simulink model "MVDRBeamformerHDLOptimizedModel"  (R2024b)
settings: Solver=FixedStepDiscrete  StartTime=0.0  StopTime=1.5  RelTol=1e-3
InitFcn:
  | % Initialize signal and noise directions
  | % https://www.mathworks.com/matlabcentral/answers/133622-how-to-change-simulink-constant-block-value-to-a-constant-variable
  | set_param([gcs,'/Noise 1 Direction'],'Value',num2str(30));
  | set_param([gcs,'/Noise 2 Direction'],'Value',num2str(50));
  | set_param([gcs,'/Signal Direction'],'Value',num2str(45));
  | set_param([gcs,'/SteeringAngle'],'Value',num2str(45));
model workspace (MAT data in the model file):
  M = 300
  OutputType : handle (value not decoded)
  T.Input = embedded.fi
  T.Input.DataType = 'Fixed'
  T.Input.Scaling = 'BinaryPoint'
  T.Input.Signed = 1
  T.Input.WordLength = 37
  T.Input.FixedExponent = -24
  T.Input.SlopeAdjustmentFactor = 1
  T.Input.Bias = 0
  T.Input.DataTypeOverride = 'Inherit'
  T.Input.intarray = [0; 0]
  T.Input.noverflows = 0
  T.Input.nunderflows = 0
  T.Input.maxlog = -1.79769313486e+308
  T.Input.minlog = 1.79769313486e+308
  T.Input.RoundingMethod = 'Nearest'
  T.Input.OverflowAction = 'Saturate'
  T.Input.ProductMode = 'FullPrecision'
  T.Input.SumMode = 'FullPrecision'
  T.Input.ProductWordLength = 32
  T.Input.SumWordLength = 32
  T.Input.MaxProductWordLength = 65535
  T.Input.MaxSumWordLength = 65535
  T.Input.ProductFractionLength = 30
  T.Input.ProductFixedExponent = -30
  T.Input.ProductSlope = 9.31322574615e-10
  T.Input.ProductSlopeAdjustmentFactor = 1
  T.Input.ProductBias = 0
  T.Input.SumFractionLength = 30
  T.Input.SumFixedExponent = -30
  T.Input.SumSlope = 9.31322574615e-10
  T.Input.SumSlopeAdjustmentFactor = 1
  T.Input.SumBias = 0
  T.Input.CastBeforeSum = 1
  T.Input.DDGMaxProductWordLength = 65535
  T.Input.DDGMaxSumWordLength = 65535
  T.Input.DDGProductFixedExponent = -30
  T.Input.DDGProductFractionLength = 30
  T.Input.DDGProductWordLength = 32
  T.Input.DDGSumFixedExponent = -30
  T.Input.DDGSumFractionLength = 30
  T.Input.DDGSumWordLength = 32
  T.Input.DDGCastBeforeSum = 1
  T.Input.DDGProductBias = 0
  T.Input.DDGProductSlopeAdjustmentFactor = 1
  T.Input.DDGSumBias = 0
  T.Input.DDGSumSlopeAdjustmentFactor = 1
  T.Input.DDGProductSlope = 9.31322574615e-10
  T.Input.DDGSumSlope = 9.31322574615e-10
  T.Input.Logging = 0
  T.Input.fimathislocal = 0
  T.Output = embedded.fi
  T.Output.DataType = 'Fixed'
  T.Output.Scaling = 'BinaryPoint'
  T.Output.Signed = 1
  T.Output.WordLength = 40
  T.Output.FixedExponent = -24
  T.Output.SlopeAdjustmentFactor = 1
  T.Output.Bias = 0
  T.Output.DataTypeOverride = 'Inherit'
  T.Output.intarray = [0; 0]
  T.Output.noverflows = 0
  T.Output.nunderflows = 0
  T.Output.maxlog = -1.79769313486e+308
  T.Output.minlog = 1.79769313486e+308
  T.Output.RoundingMethod = 'Nearest'
  T.Output.OverflowAction = 'Saturate'
  T.Output.ProductMode = 'FullPrecision'
  T.Output.SumMode = 'FullPrecision'
  T.Output.ProductWordLength = 32
  T.Output.SumWordLength = 32
  T.Output.MaxProductWordLength = 65535
  T.Output.MaxSumWordLength = 65535
  T.Output.ProductFractionLength = 30
  T.Output.ProductFixedExponent = -30
  T.Output.ProductSlope = 9.31322574615e-10
  T.Output.ProductSlopeAdjustmentFactor = 1
  T.Output.ProductBias = 0
  T.Output.SumFractionLength = 30
  T.Output.SumFixedExponent = -30
  T.Output.SumSlope = 9.31322574615e-10
  T.Output.SumSlopeAdjustmentFactor = 1
  T.Output.SumBias = 0
  T.Output.CastBeforeSum = 1
  T.Output.DDGMaxProductWordLength = 65535
  T.Output.DDGMaxSumWordLength = 65535
  T.Output.DDGProductFixedExponent = -30
  T.Output.DDGProductFractionLength = 30
  T.Output.DDGProductWordLength = 32
  T.Output.DDGSumFixedExponent = -30
  T.Output.DDGSumFractionLength = 30
  T.Output.DDGSumWordLength = 32
  T.Output.DDGCastBeforeSum = 1
  T.Output.DDGProductBias = 0
  T.Output.DDGProductSlopeAdjustmentFactor = 1
  T.Output.DDGSumBias = 0
  T.Output.DDGSumSlopeAdjustmentFactor = 1
  T.Output.DDGProductSlope = 9.31322574615e-10
  T.Output.DDGSumSlope = 9.31322574615e-10
  T.Output.Logging = 0
  T.Output.fimathislocal = 0
  T.SteeringVector = embedded.fi
  T.SteeringVector.DataType = 'Fixed'
  T.SteeringVector.Scaling = 'BinaryPoint'
  T.SteeringVector.Signed = 1
  T.SteeringVector.WordLength = 37
  T.SteeringVector.FixedExponent = -35
  T.SteeringVector.SlopeAdjustmentFactor = 1
  T.SteeringVector.Bias = 0
  T.SteeringVector.DataTypeOverride = 'Inherit'
  T.SteeringVector.intarray = [0; 0]
  T.SteeringVector.noverflows = 0
  T.SteeringVector.nunderflows = 0
  T.SteeringVector.maxlog = -1.79769313486e+308
  T.SteeringVector.minlog = 1.79769313486e+308
  T.SteeringVector.RoundingMethod = 'Floor'
  T.SteeringVector.OverflowAction = 'Wrap'
  T.SteeringVector.ProductMode = 'FullPrecision'
  T.SteeringVector.SumMode = 'FullPrecision'
  T.SteeringVector.ProductWordLength = 32
  T.SteeringVector.SumWordLength = 32
  T.SteeringVector.MaxProductWordLength = 65535
  T.SteeringVector.MaxSumWordLength = 65535
  T.SteeringVector.ProductFractionLength = 30
  T.SteeringVector.ProductFixedExponent = -30
  T.SteeringVector.ProductSlope = 9.31322574615e-10
  T.SteeringVector.ProductSlopeAdjustmentFactor = 1
  T.SteeringVector.ProductBias = 0
  T.SteeringVector.SumFractionLength = 30
  T.SteeringVector.SumFixedExponent = -30
  T.SteeringVector.SumSlope = 9.31322574615e-10
  T.SteeringVector.SumSlopeAdjustmentFactor = 1
  T.SteeringVector.SumBias = 0
  T.SteeringVector.CastBeforeSum = 1
  T.SteeringVector.DDGMaxProductWordLength = 65535
  T.SteeringVector.DDGMaxSumWordLength = 65535
  T.SteeringVector.DDGProductFixedExponent = -30
  T.SteeringVector.DDGProductFractionLength = 30
  T.SteeringVector.DDGProductWordLength = 32
  T.SteeringVector.DDGSumFixedExponent = -30
  T.SteeringVector.DDGSumFractionLength = 30
  T.SteeringVector.DDGSumWordLength = 32
  T.SteeringVector.DDGCastBeforeSum = 1
  T.SteeringVector.DDGProductBias = 0
  T.SteeringVector.DDGProductSlopeAdjustmentFactor = 1
  T.SteeringVector.DDGSumBias = 0
  T.SteeringVector.DDGSumSlopeAdjustmentFactor = 1
  T.SteeringVector.DDGProductSlope = 9.31322574615e-10
  T.SteeringVector.DDGSumSlope = 9.31322574615e-10
  T.SteeringVector.Logging = 0
  T.SteeringVector.fimathislocal = 1
  T.ForgettingFactor = embedded.fi
  T.ForgettingFactor.DataType = 'Fixed'
  T.ForgettingFactor.Scaling = 'BinaryPoint'
  T.ForgettingFactor.Signed = 1
  T.ForgettingFactor.WordLength = 37
  T.ForgettingFactor.FixedExponent = -36
  T.ForgettingFactor.SlopeAdjustmentFactor = 1
  T.ForgettingFactor.Bias = 0
  T.ForgettingFactor.DataTypeOverride = 'Inherit'
  T.ForgettingFactor.intarray = [4180530225; 15]
  T.ForgettingFactor.noverflows = 0
  T.ForgettingFactor.nunderflows = 0
  T.ForgettingFactor.maxlog = -1.79769313486e+308
  T.ForgettingFactor.minlog = 1.79769313486e+308
  T.ForgettingFactor.RoundingMethod = 'Nearest'
  T.ForgettingFactor.OverflowAction = 'Saturate'
  T.ForgettingFactor.ProductMode = 'FullPrecision'
  T.ForgettingFactor.SumMode = 'FullPrecision'
  T.ForgettingFactor.ProductWordLength = 32
  T.ForgettingFactor.SumWordLength = 32
  T.ForgettingFactor.MaxProductWordLength = 65535
  T.ForgettingFactor.MaxSumWordLength = 65535
  T.ForgettingFactor.ProductFractionLength = 30
  T.ForgettingFactor.ProductFixedExponent = -30
  T.ForgettingFactor.ProductSlope = 9.31322574615e-10
  T.ForgettingFactor.ProductSlopeAdjustmentFactor = 1
  T.ForgettingFactor.ProductBias = 0
  T.ForgettingFactor.SumFractionLength = 30
  T.ForgettingFactor.SumFixedExponent = -30
  T.ForgettingFactor.SumSlope = 9.31322574615e-10
  T.ForgettingFactor.SumSlopeAdjustmentFactor = 1
  T.ForgettingFactor.SumBias = 0
  T.ForgettingFactor.CastBeforeSum = 1
  T.ForgettingFactor.DDGMaxProductWordLength = 65535
  T.ForgettingFactor.DDGMaxSumWordLength = 65535
  T.ForgettingFactor.DDGProductFixedExponent = -30
  T.ForgettingFactor.DDGProductFractionLength = 30
  T.ForgettingFactor.DDGProductWordLength = 32
  T.ForgettingFactor.DDGSumFixedExponent = -30
  T.ForgettingFactor.DDGSumFractionLength = 30
  T.ForgettingFactor.DDGSumWordLength = 32
  T.ForgettingFactor.DDGCastBeforeSum = 1
  T.ForgettingFactor.DDGProductBias = 0
  T.ForgettingFactor.DDGProductSlopeAdjustmentFactor = 1
  T.ForgettingFactor.DDGSumBias = 0
  T.ForgettingFactor.DDGSumSlopeAdjustmentFactor = 1
  T.ForgettingFactor.DDGProductSlope = 9.31322574615e-10
  T.ForgettingFactor.DDGSumSlope = 9.31322574615e-10
  T.ForgettingFactor.Logging = 0
  T.ForgettingFactor.fimathislocal = 0
  T.M = 300
  forgettingFactor = embedded.fi
  forgettingFactor.DataType = 'Fixed'
  forgettingFactor.Scaling = 'BinaryPoint'
  forgettingFactor.Signed = 1
  forgettingFactor.WordLength = 37
  forgettingFactor.FixedExponent = -36
  forgettingFactor.SlopeAdjustmentFactor = 1
  forgettingFactor.Bias = 0
  forgettingFactor.DataTypeOverride = 'Inherit'
  forgettingFactor.intarray = [4180530225; 15]
  forgettingFactor.noverflows = 0
  forgettingFactor.nunderflows = 0
  forgettingFactor.maxlog = -1.79769313486e+308
  forgettingFactor.minlog = 1.79769313486e+308
  forgettingFactor.RoundingMethod = 'Nearest'
  forgettingFactor.OverflowAction = 'Saturate'
  forgettingFactor.ProductMode = 'FullPrecision'
  forgettingFactor.SumMode = 'FullPrecision'
  forgettingFactor.ProductWordLength = 32
  forgettingFactor.SumWordLength = 32
  forgettingFactor.MaxProductWordLength = 65535
  forgettingFactor.MaxSumWordLength = 65535
  forgettingFactor.ProductFractionLength = 30
  forgettingFactor.ProductFixedExponent = -30
  forgettingFactor.ProductSlope = 9.31322574615e-10
  forgettingFactor.ProductSlopeAdjustmentFactor = 1
  forgettingFactor.ProductBias = 0
  forgettingFactor.SumFractionLength = 30
  forgettingFactor.SumFixedExponent = -30
  forgettingFactor.SumSlope = 9.31322574615e-10
  forgettingFactor.SumSlopeAdjustmentFactor = 1
  forgettingFactor.SumBias = 0
  forgettingFactor.CastBeforeSum = 1
  forgettingFactor.DDGMaxProductWordLength = 65535
  forgettingFactor.DDGMaxSumWordLength = 65535
  forgettingFactor.DDGProductFixedExponent = -30
  forgettingFactor.DDGProductFractionLength = 30
  forgettingFactor.DDGProductWordLength = 32
  forgettingFactor.DDGSumFixedExponent = -30
  forgettingFactor.DDGSumFractionLength = 30
  forgettingFactor.DDGSumWordLength = 32
  forgettingFactor.DDGCastBeforeSum = 1
  forgettingFactor.DDGProductBias = 0
  forgettingFactor.DDGProductSlopeAdjustmentFactor = 1
  forgettingFactor.DDGSumBias = 0
  forgettingFactor.DDGSumSlopeAdjustmentFactor = 1
  forgettingFactor.DDGProductSlope = 9.31322574615e-10
  forgettingFactor.DDGSumSlope = 9.31322574615e-10
  forgettingFactor.Logging = 0
  forgettingFactor.fimathislocal = 0
  nArrayElements = 10
  noise1Variance = 100
  noise2Variance = 100
  paramBeamformerI.propSpeed = 299792458
  paramBeamformerI.fc = 100000000
  paramBeamformerI.Antenna = phased.ULA
  paramBeamformerI.Antenna.any.ClassNameForLoadTimeEval = 'phased.ULA'
  paramBeamformerI.Antenna.any.MajorVersionNumber = 24
  paramBeamformerI.Antenna.any.MinorVersionNumber = 512
  paramBeamformerI.Antenna.any.ChildClassData.NumElements = 10
  paramBeamformerI.Antenna.any.ChildClassData.ElementSpacing = 1.49896229
  paramBeamformerI.Antenna.any.ChildClassData.ArrayAxis = 'y'
  paramBeamformerI.Antenna.any.ChildClassData.Taper = 1
  paramBeamformerI.Antenna.any.ChildClassData.Element.ClassNameForLoadTimeEval = 'phased.IsotropicAntennaElement'
  paramBeamformerI.Antenna.any.ChildClassData.Element.MajorVersionNumber = 24
  paramBeamformerI.Antenna.any.ChildClassData.Element.MinorVersionNumber = 512
  paramBeamformerI.Antenna.any.ChildClassData.Element.ChildClassData.FrequencyRange = [0 1e+20]
  paramBeamformerI.Antenna.any.ChildClassData.Element.ChildClassData.BackBaffled = 0
  paramBeamformerI.Antenna.any.ChildClassData.Element.ChildClassData.pOutputCombinedPattern = 0
  paramBeamformerI.Antenna.any.ChildClassData.Element.ChildClassData.pIsOutputComplex = 1
  paramBeamformerI.Antenna.any.ChildClassData.Element.SuperClassData = []
  paramBeamformerI.Antenna.any.ChildClassData.isLocked = 0
  paramBeamformerI.Antenna.any.SuperClassData = []
  paramBeamformerI.fs = 1000
  paramBeamformerI.prf = 3.33333333333
  paramBeamformerI.samplesPerFrame = 1
  paramBeamformerI.cMatrix = [-0.976602248144+0.21505359546i  -0.840977704306+0.541069774485i  -0.61019358433+0.792252352248i; 0.347607244607-0.937640231377i  0.0788545425829-0.996886132472i  -0.186572596413-0.982441177001i; 0.600409925306+0.799692391857i  0.745453332383+0.666557821377i  0.858147047038+0.513403979006i; -0.997391183118+0.0721860640226i  -0.981896511259+0.189418164855i  -0.953897847357+0.300131465873i; 0.479000563904-0.877814593055i  0.444015840326-0.896018935927i  0.409575431342-0.912276255331i; 0.479000563904+0.877814593055i  0.444015840326+0.896018935927i  0.409575431342+0.912276255331i; -0.997391183118-0.0721860640226i  -0.981896511259-0.189418164855i  -0.953897847357-0.300131465873i; 0.600409925306-0.799692391857i  0.745453332383-0.666557821377i  0.858147047038-0.513403979006i; 0.347607244607+0.937640231377i  0.0788545425829+0.996886132472i  -0.186572596413+0.982441177001i; -0.976602248144-0.21505359546i  -0.840977704306-0.541069774485i  -0.61019358433-0.792252352248i]
  pulseMagnitude = 1
  qlessQRCyclesToReady = 46
  samplesPerFrame = 300
  thermalNoisePower = 1e-05
values from neighbouring files (symbols this model uses):
  paramBeamformerI = beamformerParameters(nArrayElements)    [setMVDRExampleModelWorkspace.m]
  T = mvdr_types('Fixed',m,nArrayElements,pulseMagnitude,thermalNoisePower,noise1Variance,noise2Variance)    [setMVDRExampleModelWorkspace.m]
undefined symbols (not defined in the file or in its folder): physconst
libraries: dspsigops x5, phasedtxrxlib x3, dspobslib x2, embsystolicmatrixops x1, embreciprocals x1, phasedwavlib x1
settings Model: DataTypeOverride=Off  SimulationMode=accelerator  Creator=The MathWorks, Inc.  LastModifiedBy=The MathWorks, Inc.
settings SolverCC: AlgebraicLoopSolver=TrustRegion  MaxZcPerStep=1
settings DataIOCC: SaveOutput=off  SignalLogging=off  SaveTime=off
settings OptimizationCC: BlockReduction=off  ConditionallyExecuteInputs=off  DefaultParameterBehavior=Inlined  ReuseModelBlockBuffer=off
settings DebuggingCC: AlgebraicLoopMsg=error  SingleTaskRateTransMsg=error  ParameterDowncastMsg=none  ParameterOverflowMsg=none  ParameterPrecisionLossMsg=none  ParameterTunabilityLossMsg=none  FixptConstOverflowMsg=warning  UnconnectedInputMsg=warning  UnconnectedOutputMsg=warning  UnconnectedLineMsg=warning
settings HardwareCC: ProdBitPerPointer=32  ProdBitPerSizeT=32  ProdBitPerPtrDiffT=32  ProdLargestAtomicFloat=None  ProdIntDivRoundTo=Undefined  ProdEndianess=Unspecified  ProdWordSize=32  ProdHWDeviceType=ASIC/FPGA->ASIC/FPGA  TargetBitPerLong=64  TargetBitPerPointer=64  TargetBitPerSizeT=64  TargetBitPerPtrDiffT=64  TargetLongLongMode=on  TargetIntDivRoundTo=Zero  TargetEndianess=LittleEndian  TargetWordSize=64  TargetHWDeviceType=Custom Processor->MATLAB Host Computer  ProdEqTarget=off
settings ModelReferenceCC: EnableRefExpFcnMdlSchedulingChecks=on
settings RTWCC: GPUComputeCapability=3.5  DLArmComputeVersion=19.05

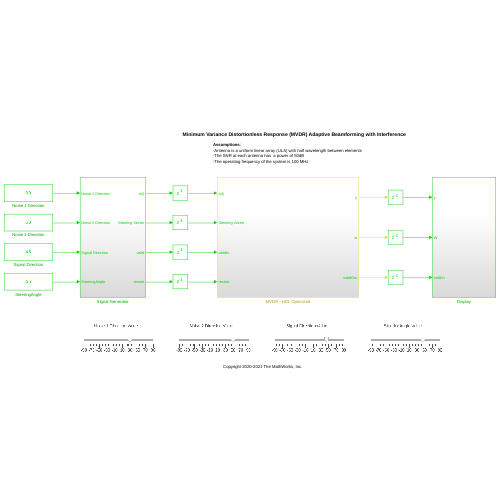
[thumbnail: Simulink's stored preview of the top-level diagram]
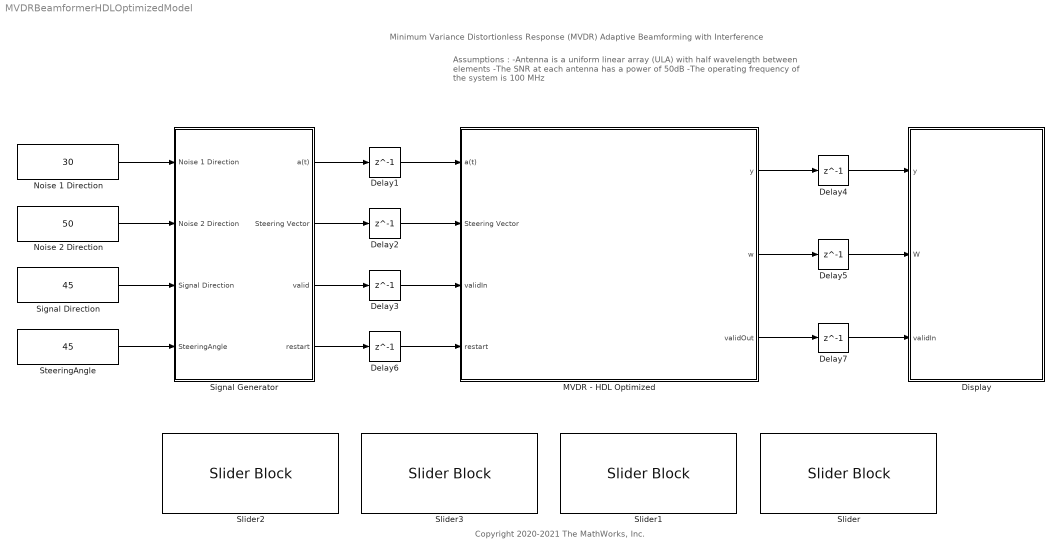
== system MVDRBeamformerHDLOptimizedModel ==
  note: Copyright 2020-2021 The MathWorks, Inc.
  note: Minimum Variance Distortionless Response (MVDR) Adaptive Beamforming with Interference
  note: Assumptions :
      | -Antenna is a uniform linear array (ULA) with half wavelength between elements
      | -The SNR at each antenna has a power of 50dB
      | -The operating frequency of the system is 100 MHz
  Delay{1..7} (7 alike) : Delay  DelayLength=1
  Display : Subsystem
  MVDR - HDL Optimized : Subsystem
  Noise 1 Direction : Constant  Value=30  VectorParams1D=off  SampleTime=-1
  Noise 2 Direction : Constant  Value=50  VectorParams1D=off  SampleTime=-1
  Signal Direction : Constant  Value=45  VectorParams1D=off  SampleTime=-1
  Signal Generator : Subsystem
  Slider{,1..3} (4 alike) : SliderBlock  ScaleMin=-90  ScaleMax=90
  SteeringAngle : Constant  Value=45  VectorParams1D=off  SampleTime=-1
  wires:
  MVDR - HDL Optimized/3(validOut) -> Delay7/1
  Delay3/1 -> MVDR - HDL Optimized/3(validIn)
  Delay4/1 -> Display/1(y)
  Signal Generator/3(valid) -> Delay3/1
  Noise 1 Direction/1 -> Signal Generator/1(Noise 1 Direction)
  Noise 2 Direction/1 -> Signal Generator/2(Noise 2 Direction)
  Signal Generator/2(Steering Vector) -> Delay2/1
  Signal Generator/4(restart) -> Delay6/1
  MVDR - HDL Optimized/1(y) -> Delay4/1
  SteeringAngle/1 -> Signal Generator/4(SteeringAngle)
  Delay5/1 -> Display/2(W)
  Signal Direction/1 -> Signal Generator/3(Signal Direction)
  MVDR - HDL Optimized/2(w) -> Delay5/1
  Delay1/1 -> MVDR - HDL Optimized/1(a(t))
  Signal Generator/1(a(t)) -> Delay1/1
  Delay2/1 -> MVDR - HDL Optimized/2(Steering Vector)
  Delay7/1 -> Display/3(validIn)
  Delay6/1 -> MVDR - HDL Optimized/4(restart)

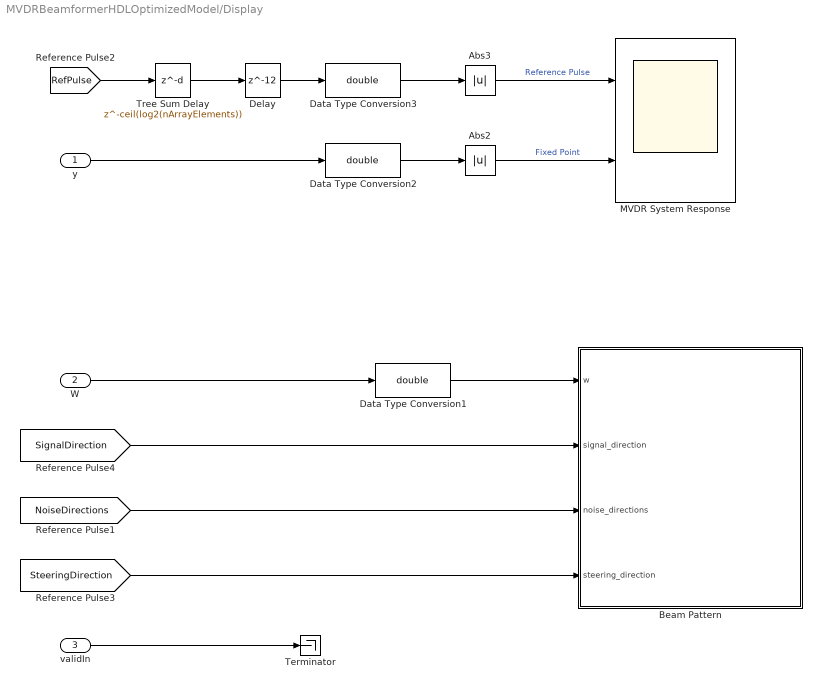
== system MVDRBeamformerHDLOptimizedModel/Display ==
  y : Inport
  W : Inport  Port=2
  validIn : Inport  Port=3
  Abs2 : Abs  SaturateOnIntegerOverflow=off
  Abs3 : Abs  SaturateOnIntegerOverflow=off
  Beam Pattern : MATLAB Function  TreatAsAtomicUnit=on  mask{M=M, nArrayElements=nArrayElements}
      mask prompts: nArrayElements "Number of array elements"
  Data Type Conversion1 : DataTypeConversion  OutDataTypeStr=double  SaturateOnIntegerOverflow=off  RndMeth=Floor
  Data Type Conversion2 : DataTypeConversion  OutDataTypeStr=double  SaturateOnIntegerOverflow=off  RndMeth=Floor
  Data Type Conversion3 : DataTypeConversion  OutDataTypeStr=double  SaturateOnIntegerOverflow=off  RndMeth=Floor
  Delay : Delay  DelayLength=12
  MVDR System Response : Scope  NumInputPorts=2
  Terminator : Terminator
  Tree Sum Delay : Delay  DelayLength=ceil(log2(nArrayElements))
  wires:
  Abs3/1 -> MVDR System Response/1  "Reference Pulse"
  Abs2/1 -> MVDR System Response/2  "Fixed Point"
  y/1 -> Data Type Conversion2/1
  Data Type Conversion2/1 -> Abs2/1
  Data Type Conversion3/1 -> Abs3/1
  [SteeringDirection] -> Beam Pattern/4(steering_direction)
  [NoiseDirections] -> Beam Pattern/3(noise_directions)
  [SignalDirection] -> Beam Pattern/2(signal_direction)
  Data Type Conversion1/1 -> Beam Pattern/1(w)
  W/1 -> Data Type Conversion1/1
  [RefPulse] -> Tree Sum Delay/1
  Delay/1 -> Data Type Conversion3/1
  validIn/1 -> Terminator/1
  Tree Sum Delay/1 -> Delay/1

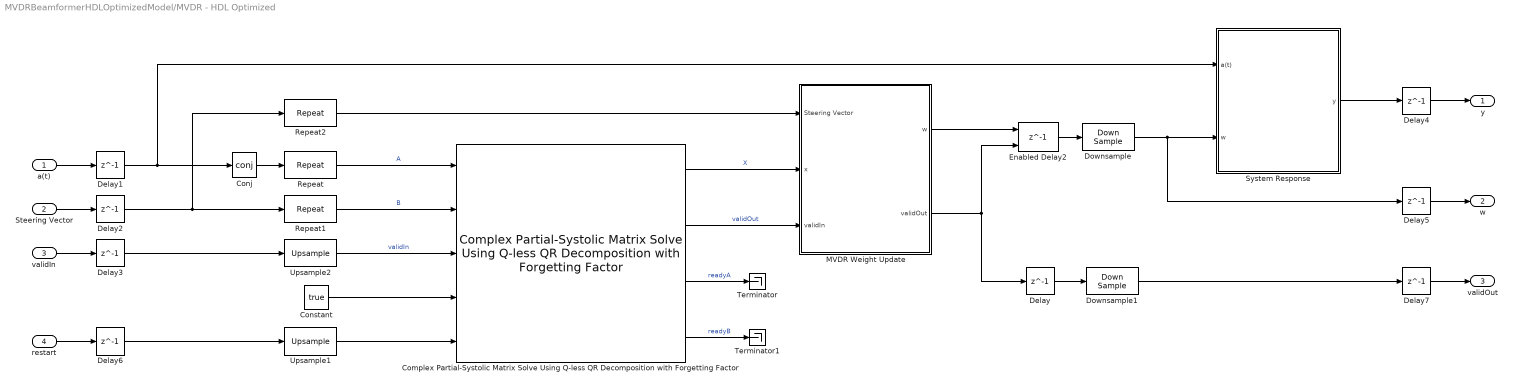
== system MVDRBeamformerHDLOptimizedModel/MVDR - HDL Optimized ==
  a(t) : Inport
  Steering Vector : Inport  Port=2
  validIn : Inport  Port=3
  restart : Inport  Port=4
  Complex Partial-Systolic Matrix Solve Using Q-less QR Decomposition with Forgetting Factor : embsystolicmatrixops/Complex Partial-Systolic Matrix Solve Using Q-less QR Decomposition with Forgetting Factor  n=nArrayElements  p=1  forgettingFactor=forgettingFactor  regularizationParameter=0  OutputType=OutputType
  Conj : Math  Operator=conj
  Constant : Constant  Value=true  OutDataTypeStr=boolean  SampleTime=-1
  Delay{,1..7} (8 alike) : Delay  DelayLength=1
  Downsample : DownSample  N=qlessQRCyclesToReady  RateOptions=Allow multirate processing
  Downsample1 : DownSample  N=qlessQRCyclesToReady  RateOptions=Allow multirate processing
  Enabled Delay2 : Delay  DelayLength=1  ShowEnablePort=on
      settings: InputPortMap=u0,e6
  MVDR Weight Update : Subsystem
  Repeat : dspsigops/Repeat  FactorSource=Dialog parameter  N=qlessQRCyclesToReady  Nmax=16  RateOptions=Allow multirate processing  ic=0  mode=Unused parameter value
  Repeat1 : dspsigops/Repeat  FactorSource=Dialog parameter  N=qlessQRCyclesToReady  Nmax=16  RateOptions=Allow multirate processing  ic=0  mode=Unused parameter value
  Repeat2 : dspsigops/Repeat  FactorSource=Dialog parameter  N=qlessQRCyclesToReady  Nmax=16  RateOptions=Allow multirate processing  ic=0  mode=Unused parameter value
  System Response : Subsystem
  Terminator : Terminator
  Terminator1 : Terminator
  Upsample1 : dspsigops/Upsample  FactorSource=Dialog parameter  N=qlessQRCyclesToReady  Nmax=16  phase=0  RateOptions=Allow multirate processing  ic=0  mode=Unused parameter value
  Upsample2 : dspsigops/Upsample  FactorSource=Dialog parameter  N=qlessQRCyclesToReady  Nmax=16  phase=0  RateOptions=Allow multirate processing  ic=0  mode=Unused parameter value
  y : Outport
  w : Outport  Port=2
  validOut : Outport  Port=3
  wires:
  System Response/1(y) -> Delay4/1
  Steering Vector/1 -> Delay2/1
  MVDR Weight Update/2(validOut) -> Delay/1, Enabled Delay2/2
  Complex Partial-Systolic Matrix Solve Using Q-less QR Decomposition with Forgetting Factor/4 -> Terminator1/1  "readyB"
  Complex Partial-Systolic Matrix Solve Using Q-less QR Decomposition with Forgetting Factor/1 -> MVDR Weight Update/2(x)  "X"
  Conj/1 -> Repeat/1
  Delay3/1 -> Upsample2/1
  MVDR Weight Update/1(w) -> Enabled Delay2/1
  Repeat1/1 -> Complex Partial-Systolic Matrix Solve Using Q-less QR Decomposition with Forgetting Factor/2  "B"
  Repeat/1 -> Complex Partial-Systolic Matrix Solve Using Q-less QR Decomposition with Forgetting Factor/1  "A"
  a(t)/1 -> Delay1/1
  validIn/1 -> Delay3/1
  Complex Partial-Systolic Matrix Solve Using Q-less QR Decomposition with Forgetting Factor/3 -> Terminator/1  "readyA"
  Upsample2/1 -> Complex Partial-Systolic Matrix Solve Using Q-less QR Decomposition with Forgetting Factor/3  "validIn"
  Delay2/1 -> Repeat2/1, Repeat1/1
  Delay4/1 -> y/1
  Delay5/1 -> w/1
  Repeat2/1 -> MVDR Weight Update/1(Steering Vector)
  Delay1/1 -> System Response/1(a(t)), Conj/1
  Enabled Delay2/1 -> Downsample/1
  Downsample/1 -> System Response/2(w), Delay5/1
  restart/1 -> Delay6/1
  Delay6/1 -> Upsample1/1
  Upsample1/1 -> Complex Partial-Systolic Matrix Solve Using Q-less QR Decomposition with Forgetting Factor/5
  Downsample1/1 -> Delay7/1
  Complex Partial-Systolic Matrix Solve Using Q-less QR Decomposition with Forgetting Factor/2 -> MVDR Weight Update/3(validIn)  "validOut"
  Delay/1 -> Downsample1/1
  Delay7/1 -> validOut/1
  Constant/1 -> Complex Partial-Systolic Matrix Solve Using Q-less QR Decomposition with Forgetting Factor/4

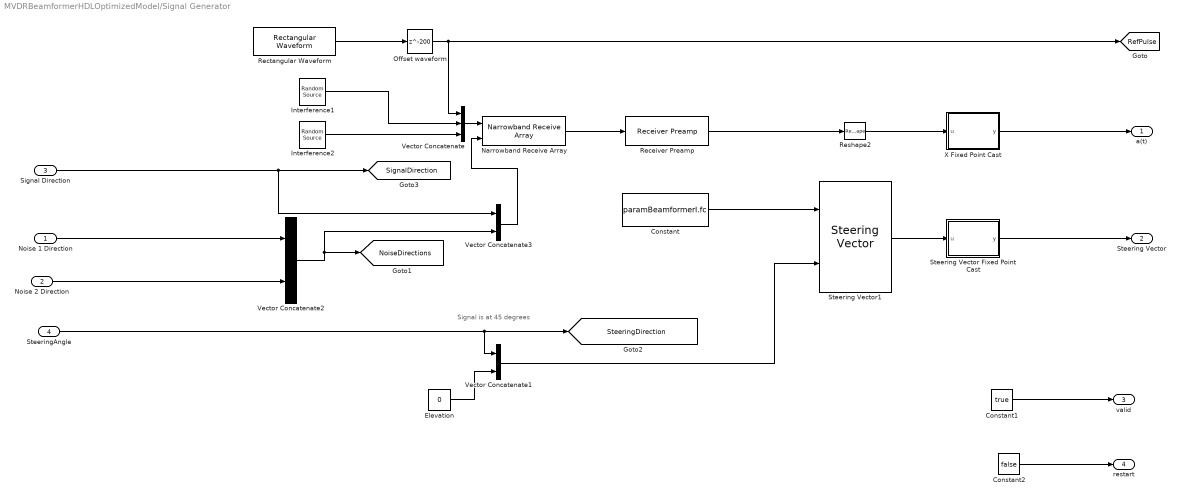
== system MVDRBeamformerHDLOptimizedModel/Signal Generator ==
  note: Signal is at 45 degrees
  Noise 1 Direction : Inport
  Noise 2 Direction : Inport  Port=2
  Signal Direction : Inport  Port=3
  SteeringAngle : Inport  Port=4
  Constant : Constant  Value=paramBeamformerI.fc
  Constant1 : Constant  Value=true  SampleTime=-1
  Constant2 : Constant  Value=false  SampleTime=-1
  Elevation : Constant  Value=0
  Interference1 : dspobslib/Random Source  SrcType=Gaussian  NormMethod=Ziggurat  CltLength=12  MinVal=0  MaxVal=1  MeanVal=0  VarVal=noise1Variance  RepMode=Repeatable  rawSeed=1  IsInherit=off  SampMode=Discrete  SampTime=1/paramBeamformerI.fs  SampFrame=paramBeamformerI.samplesPerFrame  DataType=Double  OutComplex=Real  OutputFrames=on
  Interference2 : dspobslib/Random Source  SrcType=Gaussian  NormMethod=Ziggurat  CltLength=12  MinVal=0  MaxVal=1  MeanVal=0  VarVal=noise2Variance  RepMode=Repeatable  rawSeed=1  IsInherit=off  SampMode=Discrete  SampTime=1/paramBeamformerI.fs  SampFrame=paramBeamformerI.samplesPerFrame  DataType=Double  OutComplex=Real  OutputFrames=on
  Narrowband Receive Array : phasedtxrxlib/Narrowband Receive Array  PropagationSpeed=paramBeamformerI.propSpeed  OperatingFrequency=paramBeamformerI.fc  Wavefront=Plane  SensorGainMeasure=dB  Polarization=None  WeightsInputPort=off  SimulateUsing=Interpreted execution  Sensor=paramBeamformerI.Antenna
  Offset waveform : Delay  DelayLength=200  InputProcessing=Columns as channels (frame based)
  Receiver Preamp : phasedtxrxlib/Receiver Preamp  Gain=0  LossFactor=0  NoiseMethod=Noise power  NoiseFigure=0  ReferenceTemperature=290  SampleRateFromInputCheckbox=on  SampleRate=1e6  NoisePower=thermalNoisePower  EnableInputPort=off  PhaseNoiseInputPort=off  SeedSource=Auto  Seed=0  SimulateUsing=Code generation
  Rectangular Waveform : phasedwavlib/Rectangular Waveform  SampleRate=paramBeamformerI.fs  DurationSpecification=Pulse width  PulseWidth=5/paramBeamformerI.fs  DutyCycle=0.5  PRF=paramBeamformerI.prf  PRFSelectionInputPort=off  SimulationTimeSource=Derive from waveform parameters  FrequencyOffsetSource=Property  FrequencyOffset=0  OutputFormat=Samples  NumSamples=1  NumPulses=1  PRFOutputPort=off  CoefficientsOutputPort=off  SimulateUsing=Interpreted execution
  Reshape2 : Reshape  OutputDimensionality=Column vector (2-D)
  Steering Vector Fixed Point Cast : MATLAB Function  TreatAsAtomicUnit=on  mask{T=T.SteeringVector}
      mask prompts: T "Like parameter"
  Steering Vector1 : phasedtxrxlib/Steering Vector  PropagationSpeed=physconst( 'LightSpeed' )  FrequencySource=Input port  OperatingFrequency=3e8  OutputConjugate=off  NumPhaseShifterBits=0  IncludeElementResponse=off  EnablePolarization=off  SimulateUsing=Code generation  SensorArray=paramBeamformerI.Antenna
  Vector Concatenate : Concatenate  NumInputs=3  Mode=Multidimensional array  ConcatenateDimension=2
  Vector Concatenate1 : Concatenate  Mode=Multidimensional array
  Vector Concatenate2 : Concatenate  Mode=Multidimensional array  ConcatenateDimension=2
  Vector Concatenate3 : Concatenate  Mode=Multidimensional array  ConcatenateDimension=2
  X Fixed Point Cast : MATLAB Function  TreatAsAtomicUnit=on  mask{T=T.Input}
      mask prompts: T "Like parameter"
  a(t) : Outport  VectorParamsAs1DForOutWhenUnconnected=off
  Steering Vector : Outport  Port=2  VectorParamsAs1DForOutWhenUnconnected=off
  valid : Outport  Port=3  PortDimensions=1  VectorParamsAs1DForOutWhenUnconnected=off  LockScale=on
  restart : Outport  Port=4  PortDimensions=1  VectorParamsAs1DForOutWhenUnconnected=off  LockScale=on
  tag scope: NoiseDirections=global, RefPulse=global, SignalDirection=global, SteeringDirection=global
  wires:
  Vector Concatenate3/1 -> Narrowband Receive Array/2
  Interference1/1 -> Vector Concatenate/2
  Interference2/1 -> Vector Concatenate/3
  Elevation/1 -> Vector Concatenate1/2
  Vector Concatenate2/1 -> Vector Concatenate3/2, [NoiseDirections]
  Rectangular Waveform/1 -> Offset waveform/1
  Vector Concatenate/1 -> Narrowband Receive Array/1
  Offset waveform/1 -> [RefPulse], Vector Concatenate/1
  Narrowband Receive Array/1 -> Receiver Preamp/1
  Constant/1 -> Steering Vector1/1
  Vector Concatenate1/1 -> Steering Vector1/2
  Steering Vector1/1 -> Steering Vector Fixed Point Cast/1(u)
  Steering Vector Fixed Point Cast/1(y) -> Steering Vector/1
  Reshape2/1 -> X Fixed Point Cast/1(u)
  X Fixed Point Cast/1(y) -> a(t)/1
  Receiver Preamp/1 -> Reshape2/1
  Signal Direction/1 -> Vector Concatenate3/1, [SignalDirection]
  Noise 1 Direction/1 -> Vector Concatenate2/1
  Noise 2 Direction/1 -> Vector Concatenate2/2
  SteeringAngle/1 -> Vector Concatenate1/1, [SteeringDirection]
  Constant1/1 -> valid/1
  Constant2/1 -> restart/1

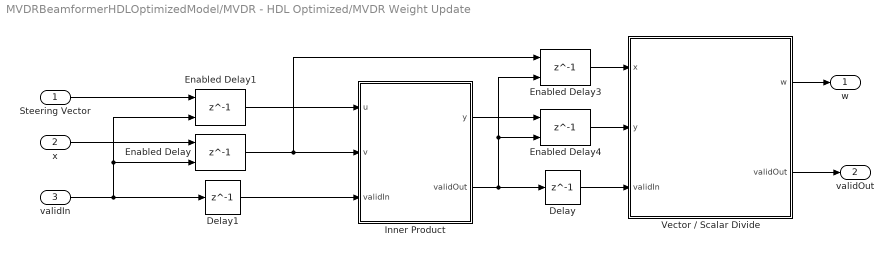
== system MVDRBeamformerHDLOptimizedModel/MVDR - HDL Optimized/MVDR Weight Update ==
  Steering Vector : Inport
  x : Inport  Port=2
  validIn : Inport  Port=3
  Delay : Delay  DelayLength=1
  Delay1 : Delay  DelayLength=1
  Enabled Delay{,1,3..4} (4 alike) : Delay  DelayLength=1  ShowEnablePort=on
      settings: InputPortMap=u0,e6
  Inner Product : Subsystem  mask{n=nArrayElements}
      mask prompts: n "Vector length"
  Vector / Scalar Divide : Subsystem
  w : Outport
  validOut : Outport  Port=2
  wires:
  x/1 -> Enabled Delay/1
  Vector / Scalar Divide/1(w) -> w/1
  Enabled Delay1/1 -> Inner Product/1(u)
  Inner Product/1(y) -> Enabled Delay4/1
  Enabled Delay3/1 -> Vector / Scalar Divide/1(x)
  Delay/1 -> Vector / Scalar Divide/3(validIn)
  Steering Vector/1 -> Enabled Delay1/1
  Enabled Delay/1 -> Enabled Delay3/1, Inner Product/2(v)
  Enabled Delay4/1 -> Vector / Scalar Divide/2(y)
  Inner Product/2(validOut) -> Enabled Delay4/2, Enabled Delay3/2, Delay/1
  validIn/1 -> Enabled Delay1/2, Enabled Delay/2, Delay1/1
  Vector / Scalar Divide/2(validOut) -> validOut/1
  Delay1/1 -> Inner Product/3(validIn)

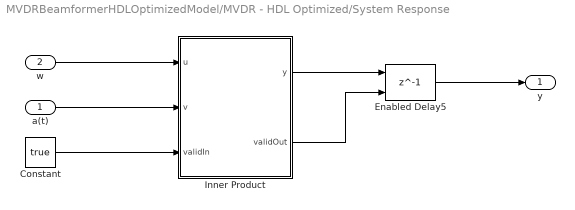
== system MVDRBeamformerHDLOptimizedModel/MVDR - HDL Optimized/System Response ==
  a(t) : Inport
  w : Inport  Port=2
  Constant : Constant  Value=true  SampleTime=-1
  Enabled Delay5 : Delay  DelayLength=1  ShowEnablePort=on
      settings: InputPortMap=u0,e6
  Inner Product : Subsystem  mask{n=nArrayElements}
      mask prompts: n "Vector length"
  y : Outport
  wires:
  Enabled Delay5/1 -> y/1
  a(t)/1 -> Inner Product/2(v)
  Inner Product/2(validOut) -> Enabled Delay5/2
  Constant/1 -> Inner Product/3(validIn)
  Inner Product/1(y) -> Enabled Delay5/1
  w/1 -> Inner Product/1(u)

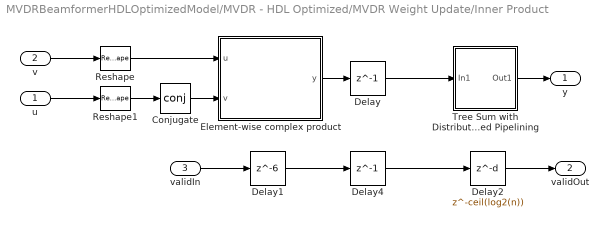
== system MVDRBeamformerHDLOptimizedModel/MVDR - HDL Optimized/MVDR Weight Update/Inner Product ==
  u : Inport
  v : Inport  Port=2
  validIn : Inport  Port=3
  Conjugate : Math  Operator=conj  SignedPower=on  RndMeth=Zero
  Delay : Delay  DelayLength=1
  Delay1 : Delay  DelayLength=6
  Delay2 : Delay  DelayLength=ceil(log2(n))
  Delay4 : Delay  DelayLength=1
  Element-wise complex product : Subsystem  TreatAsAtomicUnit=on
  Reshape : Reshape  OutputDimensionality=Column vector (2-D)
  Reshape1 : Reshape  OutputDimensionality=Column vector (2-D)
  Tree Sum with Distributed Pipelining : Subsystem
  y : Outport
  validOut : Outport  Port=2
  wires:
  v/1 -> Reshape/1
  u/1 -> Reshape1/1
  validIn/1 -> Delay1/1
  Element-wise complex product/1(y) -> Delay/1
  Delay2/1 -> validOut/1
  Delay1/1 -> Delay4/1
  Delay4/1 -> Delay2/1
  Reshape/1 -> Element-wise complex product/1(u)
  Delay/1 -> Tree Sum with Distributed Pipelining/1(In1)
  Tree Sum with Distributed Pipelining/1(Out1) -> y/1
  Reshape1/1 -> Conjugate/1
  Conjugate/1 -> Element-wise complex product/2(v)

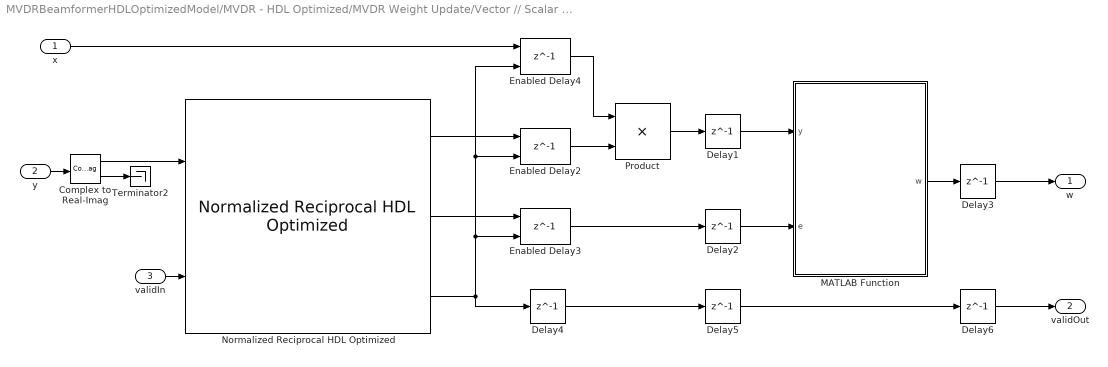
== system MVDRBeamformerHDLOptimizedModel/MVDR - HDL Optimized/MVDR Weight Update/Vector // Scalar Divide ==
  x : Inport
  y : Inport  Port=2
  validIn : Inport  Port=3
  Complex to Real-Imag : ComplexToRealImag
  Delay{1..6} (6 alike) : Delay  DelayLength=1
  Enabled Delay2 : Delay  DelayLength=1  ShowEnablePort=on
      settings: InputPortMap=u0,e6
  Enabled Delay3 : Delay  DelayLength=1  ShowEnablePort=on
      settings: InputPortMap=u0,e6
  Enabled Delay4 : Delay  DelayLength=1  ShowEnablePort=on
      settings: InputPortMap=u0,e6
  MATLAB Function : MATLAB Function  TreatAsAtomicUnit=on
  Normalized Reciprocal HDL Optimized : embreciprocals/Normalized Reciprocal HDL Optimized  dbzPort=off  autoMaximumShiftVal=on  maximumShiftValue=10  nIterPerReg=1
  Product : Product  OutDataTypeStr=Inherit: Same as first input
  Terminator2 : Terminator
  w : Outport
  validOut : Outport  Port=2
  wires:
  Delay2/1 -> MATLAB Function/2(e)
  y/1 -> Complex to Real-Imag/1
  Enabled Delay2/1 -> Product/2
  Complex to Real-Imag/1 -> Normalized Reciprocal HDL Optimized/1
  Enabled Delay4/1 -> Product/1
  Normalized Reciprocal HDL Optimized/2 -> Enabled Delay3/1
  Normalized Reciprocal HDL Optimized/1 -> Enabled Delay2/1
  Delay1/1 -> MATLAB Function/1(y)
  validIn/1 -> Normalized Reciprocal HDL Optimized/2
  Product/1 -> Delay1/1
  Enabled Delay3/1 -> Delay2/1
  MATLAB Function/1(w) -> Delay3/1
  Complex to Real-Imag/2 -> Terminator2/1
  x/1 -> Enabled Delay4/1
  Normalized Reciprocal HDL Optimized/3 -> Delay4/1, Enabled Delay3/2, Enabled Delay4/2, Enabled Delay2/2
  Delay3/1 -> w/1
  Delay4/1 -> Delay5/1
  Delay5/1 -> Delay6/1
  Delay6/1 -> validOut/1

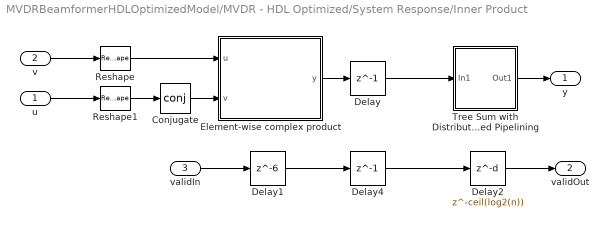
== system MVDRBeamformerHDLOptimizedModel/MVDR - HDL Optimized/System Response/Inner Product ==
  u : Inport
  v : Inport  Port=2
  validIn : Inport  Port=3
  Conjugate : Math  Operator=conj  SignedPower=on  RndMeth=Zero
  Delay : Delay  DelayLength=1
  Delay1 : Delay  DelayLength=6
  Delay2 : Delay  DelayLength=ceil(log2(n))
  Delay4 : Delay  DelayLength=1
  Element-wise complex product : Subsystem  TreatAsAtomicUnit=on
  Reshape : Reshape  OutputDimensionality=Column vector (2-D)
  Reshape1 : Reshape  OutputDimensionality=Column vector (2-D)
  Tree Sum with Distributed Pipelining : Subsystem
  y : Outport
  validOut : Outport  Port=2
  wires:
  v/1 -> Reshape/1
  u/1 -> Reshape1/1
  validIn/1 -> Delay1/1
  Element-wise complex product/1(y) -> Delay/1
  Delay2/1 -> validOut/1
  Delay1/1 -> Delay4/1
  Delay4/1 -> Delay2/1
  Reshape/1 -> Element-wise complex product/1(u)
  Delay/1 -> Tree Sum with Distributed Pipelining/1(In1)
  Tree Sum with Distributed Pipelining/1(Out1) -> y/1
  Reshape1/1 -> Conjugate/1
  Conjugate/1 -> Element-wise complex product/2(v)

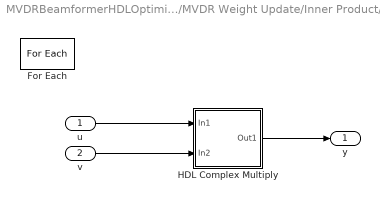
== system MVDRBeamformerHDLOptimizedModel/MVDR - HDL Optimized/MVDR Weight Update/Inner Product/Element-wise complex product ==
  u : Inport  Partition=on  PartitionDimension=1  PartitionWidth=1  PartitionOffset=0
  v : Inport  Port=2  Partition=on  PartitionDimension=1  PartitionWidth=1  PartitionOffset=0
  For Each : ForEach  DisableCoverage=on
  HDL Complex Multiply : Subsystem  mask(HDL Complex Multiplier (3 Multiply, 5 Add)){D1=2, D2=1, D3=1, D4=1, D5=1}
      mask help:
      | Xilinx devices:
      | - Set D1 = 1 or 2 to trade off speed & FF resources
      | - Set D2-D5 = 1 to fully leverage DSP48 pipelines
      | - Use sync reset
      |
      | Intel FPGAs:
      | - Set D1 = 1 or 2 depending on device family
      | - Set D5 = 1; D2, D3, D4 = 0
      | - Use async reset
      mask init:
      | delay = D1+D2+D3+D4+D5;
      mask Display:
      | fprintf('Delay=%d',delay);
      | port_label('input',1,'z1');
      | port_label('input',2,'z2');
  y : Outport  ConcatenationDimension=1
  wires:
  v/1 -> HDL Complex Multiply/2(In2)
  HDL Complex Multiply/1(Out1) -> y/1
  u/1 -> HDL Complex Multiply/1(In1)

== system MVDRBeamformerHDLOptimizedModel/MVDR - HDL Optimized/MVDR Weight Update/Inner Product/Tree Sum with Distributed Pipelining ==
  In1 : Inport
  Delay3 : Delay  DelayLength=ceil(log2(n))
  Tree Sum of Elements : Sum  Inputs=+  OutDataTypeStr=Inherit: Same as first input  LockScale=on
  Out1 : Outport
  wires:
  Delay3/1 -> Out1/1
  In1/1 -> Tree Sum of Elements/1
  Tree Sum of Elements/1 -> Delay3/1

== system MVDRBeamformerHDLOptimizedModel/MVDR - HDL Optimized/System Response/Inner Product/Element-wise complex product ==
  u : Inport  Partition=on  PartitionDimension=1  PartitionWidth=1  PartitionOffset=0
  v : Inport  Port=2  Partition=on  PartitionDimension=1  PartitionWidth=1  PartitionOffset=0
  For Each : ForEach  DisableCoverage=on
  HDL Complex Multiply : Subsystem  mask(HDL Complex Multiplier (3 Multiply, 5 Add)){D1=2, D2=1, D3=1, D4=1, D5=1}
      mask help:
      | Xilinx devices:
      | - Set D1 = 1 or 2 to trade off speed & FF resources
      | - Set D2-D5 = 1 to fully leverage DSP48 pipelines
      | - Use sync reset
      |
      | Intel FPGAs:
      | - Set D1 = 1 or 2 depending on device family
      | - Set D5 = 1; D2, D3, D4 = 0
      | - Use async reset
      mask init:
      | delay = D1+D2+D3+D4+D5;
      mask Display:
      | fprintf('Delay=%d',delay);
      | port_label('input',1,'z1');
      | port_label('input',2,'z2');
  y : Outport  ConcatenationDimension=1
  wires:
  v/1 -> HDL Complex Multiply/2(In2)
  HDL Complex Multiply/1(Out1) -> y/1
  u/1 -> HDL Complex Multiply/1(In1)

== system MVDRBeamformerHDLOptimizedModel/MVDR - HDL Optimized/System Response/Inner Product/Tree Sum with Distributed Pipelining ==
  In1 : Inport
  Delay3 : Delay  DelayLength=ceil(log2(n))
  Tree Sum of Elements : Sum  Inputs=+  OutDataTypeStr=Inherit: Same as first input  LockScale=on
  Out1 : Outport
  wires:
  Delay3/1 -> Out1/1
  In1/1 -> Tree Sum of Elements/1
  Tree Sum of Elements/1 -> Delay3/1

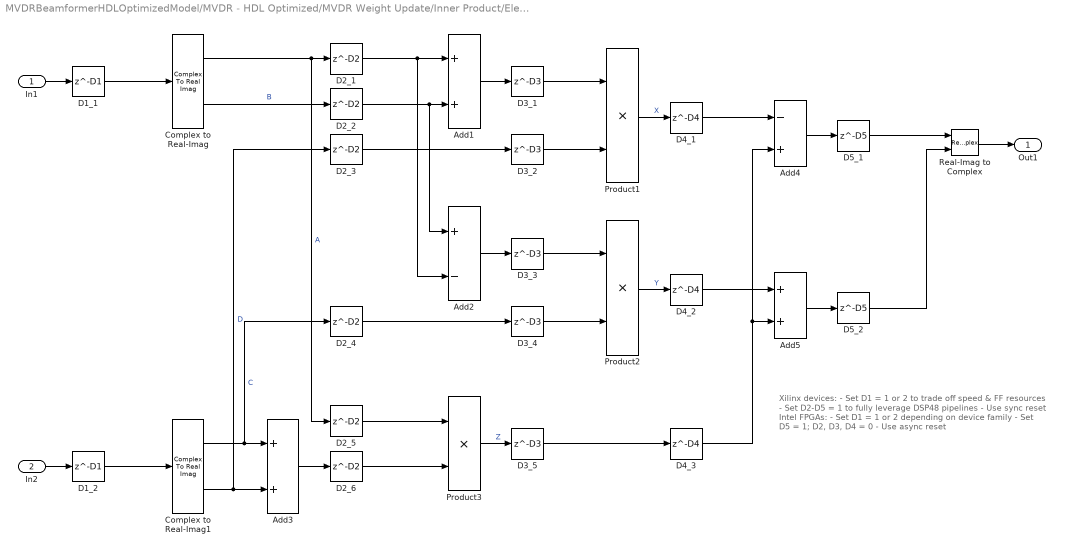
== system MVDRBeamformerHDLOptimizedModel/MVDR - HDL Optimized/MVDR Weight Update/Inner Product/Element-wise complex product/HDL Complex Multiply ==
  note: Xilinx devices:
      | - Set D1 = 1 or 2 to trade off speed & FF resources
      | - Set D2-D5 = 1 to fully leverage DSP48 pipelines
      | - Use sync reset
      |
      | Intel FPGAs:
      | - Set D1 = 1 or 2 depending on device family
      | - Set D5 = 1; D2, D3, D4 = 0
      | - Use async reset
  In1 : Inport
  In2 : Inport  Port=2
  Add1 : Sum
  Add2 : Sum  Inputs=+-
  Add3 : Sum
  Add4 : Sum  Inputs=-+
  Add5 : Sum
  Complex to Real-Imag : ComplexToRealImag
  Complex to Real-Imag1 : ComplexToRealImag
  D1_1 : Delay  DelayLength=D1
  D1_2 : Delay  DelayLength=D1
  D2_{1..6} (6 alike) : Delay  DelayLength=D2
  D3_{1..5} (5 alike) : Delay  DelayLength=D3
  D4_1 : Delay  DelayLength=D4
  D4_2 : Delay  DelayLength=D4
  D4_3 : Delay  DelayLength=D4
  D5_1 : Delay  DelayLength=D5
  D5_2 : Delay  DelayLength=D5
  Product1 : Product  OutDataTypeStr=Inherit: Same as first input
  Product2 : Product  OutDataTypeStr=Inherit: Same as first input
  Product3 : Product  OutDataTypeStr=Inherit: Same as first input
  Real-Imag to Complex : RealImagToComplex
  Out1 : Outport  VectorParamsAs1DForOutWhenUnconnected=off
  wires:
  Real-Imag to Complex/1 -> Out1/1
  In2/1 -> D1_2/1
  Complex to Real-Imag1/1 -> Add3/1, D2_4/1  "C"
  Complex to Real-Imag1/2 -> Add3/2, D2_3/1  "D"
  Product1/1 -> D4_1/1  "X"
  Product2/1 -> D4_2/1  "Y"
  Product3/1 -> D3_5/1  "Z"
  Add4/1 -> D5_1/1
  Add5/1 -> D5_2/1
  D5_1/1 -> Real-Imag to Complex/1
  D5_2/1 -> Real-Imag to Complex/2
  D4_1/1 -> Add4/1
  D4_2/1 -> Add5/1
  D3_5/1 -> D4_3/1
  Add1/1 -> D3_1/1
  Add3/1 -> D2_6/1
  Add2/1 -> D3_3/1
  Complex to Real-Imag/1 -> D2_5/1, D2_1/1  "A"
  Complex to Real-Imag/2 -> D2_2/1  "B"
  D3_1/1 -> Product1/1
  D2_6/1 -> Product3/2
  D3_3/1 -> Product2/1
  D4_3/1 -> Add4/2, Add5/2
  D3_4/1 -> Product2/2
  D3_2/1 -> Product1/2
  D2_4/1 -> D3_4/1
  D2_3/1 -> D3_2/1
  D2_5/1 -> Product3/1
  D2_2/1 -> Add1/2, Add2/1
  D2_1/1 -> Add2/2, Add1/1
  In1/1 -> D1_1/1
  D1_1/1 -> Complex to Real-Imag/1
  D1_2/1 -> Complex to Real-Imag1/1

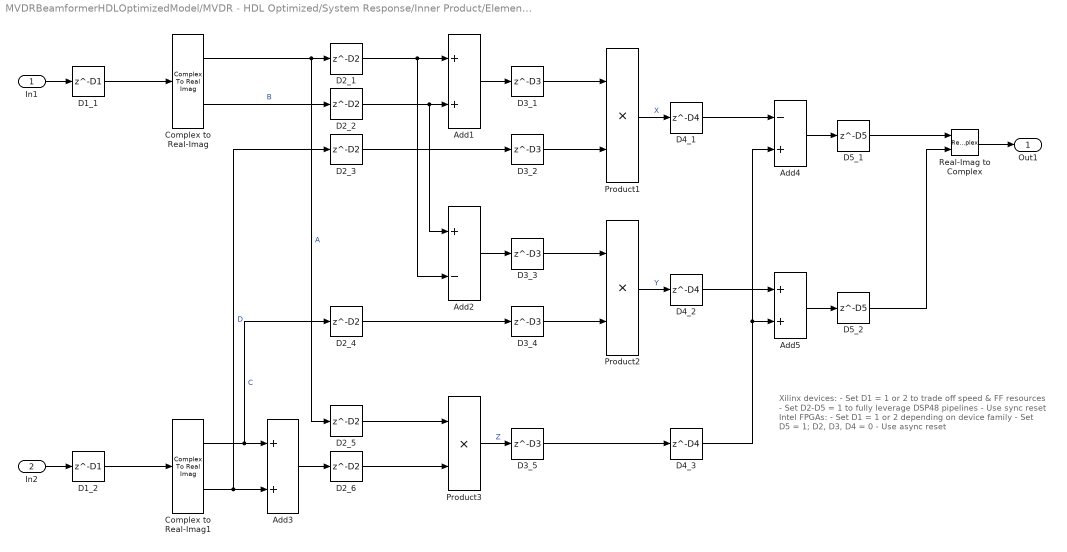
== system MVDRBeamformerHDLOptimizedModel/MVDR - HDL Optimized/System Response/Inner Product/Element-wise complex product/HDL Complex Multiply ==
  note: Xilinx devices:
      | - Set D1 = 1 or 2 to trade off speed & FF resources
      | - Set D2-D5 = 1 to fully leverage DSP48 pipelines
      | - Use sync reset
      |
      | Intel FPGAs:
      | - Set D1 = 1 or 2 depending on device family
      | - Set D5 = 1; D2, D3, D4 = 0
      | - Use async reset
  In1 : Inport
  In2 : Inport  Port=2
  Add1 : Sum
  Add2 : Sum  Inputs=+-
  Add3 : Sum
  Add4 : Sum  Inputs=-+
  Add5 : Sum
  Complex to Real-Imag : ComplexToRealImag
  Complex to Real-Imag1 : ComplexToRealImag
  D1_1 : Delay  DelayLength=D1
  D1_2 : Delay  DelayLength=D1
  D2_{1..6} (6 alike) : Delay  DelayLength=D2
  D3_{1..5} (5 alike) : Delay  DelayLength=D3
  D4_1 : Delay  DelayLength=D4
  D4_2 : Delay  DelayLength=D4
  D4_3 : Delay  DelayLength=D4
  D5_1 : Delay  DelayLength=D5
  D5_2 : Delay  DelayLength=D5
  Product1 : Product  OutDataTypeStr=Inherit: Same as first input
  Product2 : Product  OutDataTypeStr=Inherit: Same as first input
  Product3 : Product  OutDataTypeStr=Inherit: Same as first input
  Real-Imag to Complex : RealImagToComplex
  Out1 : Outport  VectorParamsAs1DForOutWhenUnconnected=off
  wires:
  Real-Imag to Complex/1 -> Out1/1
  In2/1 -> D1_2/1
  Complex to Real-Imag1/1 -> Add3/1, D2_4/1  "C"
  Complex to Real-Imag1/2 -> Add3/2, D2_3/1  "D"
  Product1/1 -> D4_1/1  "X"
  Product2/1 -> D4_2/1  "Y"
  Product3/1 -> D3_5/1  "Z"
  Add4/1 -> D5_1/1
  Add5/1 -> D5_2/1
  D5_1/1 -> Real-Imag to Complex/1
  D5_2/1 -> Real-Imag to Complex/2
  D4_1/1 -> Add4/1
  D4_2/1 -> Add5/1
  D3_5/1 -> D4_3/1
  Add1/1 -> D3_1/1
  Add3/1 -> D2_6/1
  Add2/1 -> D3_3/1
  Complex to Real-Imag/1 -> D2_5/1, D2_1/1  "A"
  Complex to Real-Imag/2 -> D2_2/1  "B"
  D3_1/1 -> Product1/1
  D2_6/1 -> Product3/2
  D3_3/1 -> Product2/1
  D4_3/1 -> Add4/2, Add5/2
  D3_4/1 -> Product2/2
  D3_2/1 -> Product1/2
  D2_4/1 -> D3_4/1
  D2_3/1 -> D3_2/1
  D2_5/1 -> Product3/1
  D2_2/1 -> Add1/2, Add2/1
  D2_1/1 -> Add2/2, Add1/1
  In1/1 -> D1_1/1
  D1_1/1 -> Complex to Real-Imag/1
  D1_2/1 -> Complex to Real-Imag1/1

== matlab function MVDRBeamformerHDLOptimizedModel/Display/Beam Pattern ==
  data: w input; signal_direction input; noise_directions input; steering_direction input; M parameter size=1; nArrayElements parameter size=1
function beamPattern(w,signal_direction,noise_directions,steering_direction,M,nArrayElements)
    coder.extrinsic('pattern');
    coder.extrinsic('axis');
    coder.extrinsic('figure');
    coder.extrinsic('drawnow');
    coder.extrinsic('phased.ULA');
    coder.extrinsic('xline');
    coder.extrinsic('yline');
    coder.extrinsic('figure');
    coder.extrinsic('gcf');
    coder.extrinsic('set');
    % Constants
    line_width = 2;
    carrierFreq = 100e6;
    wavelength = physconst('LightSpeed')/carrierFreq;
    
    % Persistent variables
    persistent fig counter
    persistent ula
    persistent pattern_line
    persistent noise1_line noise2_line
    persistent signal_line
    persistent steering_line
    if isempty(ula)
        counter = 0;
        ula = phased.ULA('NumElements',nArrayElements,'ElementSpacing',wavelength/2);
        %ula.Element.FrequencyRange = [90e5 110e6];
        fig = gcf;
        figure(fig)
        clf(fig)
        set(fig,'Name','Beam Pattern');
        [PAT,AZ_ANG,~] = pattern(ula,carrierFreq,-90:90,0,'Weights',w,'Type','powerdb',...
            'PropagationSpeed',physconst('LightSpeed'),'Normalize',false,...
            'CoordinateSystem','rectangular');
        pattern_line = line(AZ_ANG,PAT,'LineWidth',line_width);
        title('MVDR Beam Pattern')
        xlabel('Azimuth Angle (degrees)')
        ylabel('Power (dB)')
        box on
        axis([-90 90 -40 40]);
        yline(0)
        grid on
        axis on
        noise1_line = xline(noise_directions(1),'red','LineWidth',line_width);
        noise2_line = xline(noise_directions(2),'red','LineWidth',line_width);
        signal_line = xline(signal_direction,'green','LineWidth',4);
        steering_line = xline(steering_direction,'blue','LineWidth',line_width);
    end
    counter = counter + 1;
    if counter == M
        counter = 0;
        [PAT,~,~] = pattern(ula,carrierFreq,-90:90,0,'Weights',w,'Type','powerdb',...
            'PropagationSpeed',physconst('LightSpeed'),'Normalize',false,...
            'CoordinateSystem','rectangular');
        set(pattern_line,'YData',PAT);
        set(noise1_line,'Value',noise_directions(1));
        set(noise2_line,'Value',noise_directions(2));
        set(signal_line,'Value',signal_direction);
        set(steering_line,'Value',steering_direction);
        drawnow
    end
end

== matlab function MVDRBeamformerHDLOptimizedModel/MVDR - HDL Optimized/MVDR Weight Update/Vector // Scalar Divide/MATLAB Function ==
  data: y input; w output; e input
function w = variableShift(y,e)
    %#codegen
    w = fixed.bitshift(y,e);
end

== matlab function MVDRBeamformerHDLOptimizedModel/Signal Generator/Steering Vector Fixed Point Cast ==
  data: u input; y output; T parameter
function y = cast_like(u,T)
    y = cast(u,'like',T);
end

== matlab function MVDRBeamformerHDLOptimizedModel/Signal Generator/X Fixed Point Cast ==
  data: u input; y output; T parameter
function y = cast_like(u,T)
    y = cast(u,'like',T);
end
